simulink model "G_cl_circuit"  (R2020b)
settings: Solver=VariableStepAuto  StartTime=0.0  StopTime=10.0  RelTol=1e-3
undefined symbols (not defined in the file): R_s, Z_3, Z_5, Z_mot
libraries: cstblocks x4, fod x1
settings Model: Creator=jasper  LastModifiedBy=jasper

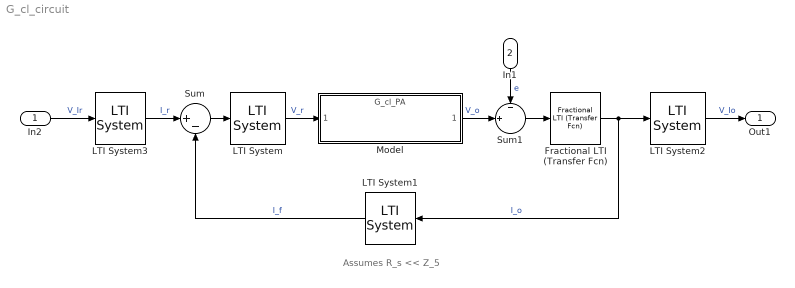
== system G_cl_circuit ==
  note: Assumes R_s << Z_5
  In2 : Inport
  In1 : Inport  Port=2
  Fractional LTI (Transfer Fcn) : fod/Fractional LTI (Transfer Fcn)  G=1/Z_mot  freqRange=[0.001 1000]  approxNum=5  useRef=off
      settings: SourceProductName=FOMCON Toolbox
  LTI System : cstblocks/LTI System  sys=Z_4  IC=[]
  LTI System1 : cstblocks/LTI System  sys=R_s/Z_5  IC=[]
  LTI System2 : cstblocks/LTI System  sys=R_s  IC=[]
  LTI System3 : cstblocks/LTI System  sys=-1/Z_3  IC=[]
  Model : ModelReference  ModelNameDialog=G_cl_PA.slx  SimulationMode=Normal  ModelReferenceVersion=1.2
  Sum : Sum  Inputs=|+-
  Sum1 : Sum  Inputs=-|+||
  Out1 : Outport
  wires:
  Sum/1 -> LTI System/1
  LTI System/1 -> Model/1  "V_r"
  Model/1 -> Sum1/2  "V_o"
  In1/1 -> Sum1/1  "e"
  Sum1/1 -> Fractional LTI (Transfer Fcn)/1
  Fractional LTI (Transfer Fcn)/1 -> LTI System2/1, LTI System1/1  "I_o"
  LTI System1/1 -> Sum/2  "I_f"
  LTI System2/1 -> Out1/1  "V_Io"
  LTI System3/1 -> Sum/1  "I_r"
  In2/1 -> LTI System3/1  "V_Ir"
